simulink model "port_test_B_2013B"  (R2013b)
settings: Solver=ode45  StartTime=0.0  StopTime=10  RelTol=1e-3
libraries: dspnetwork x4, rtwinlib x1
settings Model: CovModelRefEnable=off  Creator=dave  LastModifiedBy=Anony
settings DataIOCC: SaveFormat=StructureWithTime
settings DebuggingCC: UnderspecifiedInitializationDetection=Simplified  MergeDetectMultiDrivingBlocksExec=error  SolverPrmCheckMsg=none  FrameProcessingCompatibilityMsg=error
settings HardwareCC: ProdBitPerPointer=64  ProdLargestAtomicFloat=Float  ProdIntDivRoundTo=Zero  ProdEndianess=LittleEndian  ProdHWDeviceType=Specified
settings GRTTargetCC: CodeReplacementLibrary=C89/C90 (ANSI)  GeneratePreprocessorConditionals=Use local settings

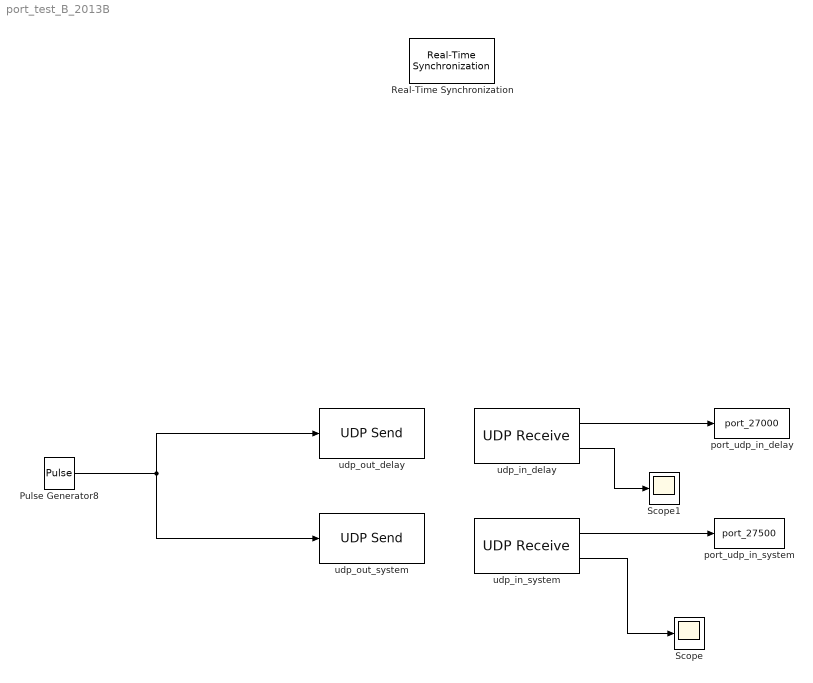
== system port_test_B_2013B ==
  Pulse Generator8 : DiscretePulseGenerator  PulseType=Time based  Period=1  PulseWidth=5
  Real-Time Synchronization : rtwinlib/Real-Time Synchronization  SampleTime=0.1  MaxMissedTicks=inf  ShowMissedTicks=off  YieldWhenWaiting=off
  Scope : Scope
      settings: TimeRange=auto  LimitDataPoints=on  MaxDataPoints=5000  SaveToWorkspace=off  SaveName=ScopeData  YMin=-10  YMax=10  SampleTime=-1  DataFormat=Array
  Scope1 : Scope
      settings: TimeRange=auto  LimitDataPoints=on  MaxDataPoints=5000  SaveToWorkspace=off  YMin=-10  YMax=10  SampleTime=-1  DataFormat=Array
  port_udp_in_delay : ToWorkspace  VariableName=port_27000  SaveFormat=Timeseries  SampleTime=-1
  port_udp_in_system : ToWorkspace  VariableName=port_27500  SaveFormat=Timeseries  SampleTime=-1
  udp_in_delay : dspnetwork/UDP Receive  localURL='0.0.0.0'  localPort=27000  remoteURL='147.32.183.0'  remotePort=-1  recvBufferSize=8192  dims=255  signalDatatype=int8  isVarSize=off  showBlockingTime=off  blockingTime=0  sampletime=0.1
  udp_in_system : dspnetwork/UDP Receive  localURL='0.0.0.0'  localPort=27500  remoteURL='147.32.183.0'  remotePort=-1  recvBufferSize=8192  dims=255  signalDatatype=int8  isVarSize=off  showBlockingTime=off  blockingTime=0  sampletime=0.1
  udp_out_delay : dspnetwork/UDP Send  remoteURL='147.32.183.0'  remotePort=28000  localURL='0.0.0.0'  localPortSource=Automatically determine  localPort=-1  sampletime=-1  separateLengthPort=0
  udp_out_system : dspnetwork/UDP Send  remoteURL='147.32.183.0'  remotePort=28500  localURL='0.0.0.0'  localPortSource=Automatically determine  localPort=-1  sampletime=-1  separateLengthPort=0
  wires:
  Pulse Generator8/1 -> udp_out_delay/1, udp_out_system/1
  udp_in_system/1 -> port_udp_in_system/1
  udp_in_delay/1 -> port_udp_in_delay/1
  udp_in_system/2 -> Scope/1
  udp_in_delay/2 -> Scope1/1
